simulink model "restart_lv1"  (Simulink 7.1)
settings: Solver=ode3  StartTime=0.0  StopTime=100  FixedStep=0.01  RelTol=1e-3
undefined symbols (not defined in the file or in its folder): fcn
libraries: DRlib x1
settings Model: Creator=lv  LastModifiedBy=lv

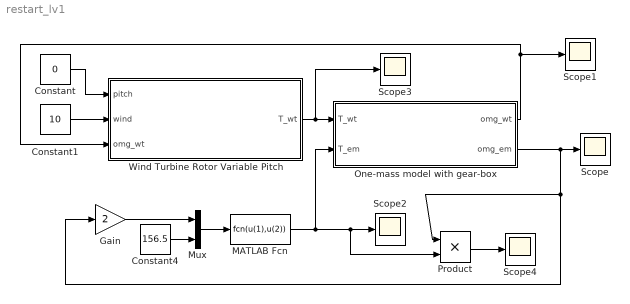
== system restart_lv1 ==
  Constant : Constant  Value=0  OutDataType=sfix(16)  OutScaling=2^0
  Constant1 : Constant  Value=10  OutDataType=sfix(16)  OutScaling=2^0
  Constant4 : Constant  Value=156.5  OutDataType=sfix(16)  OutScaling=2^0
  Gain : Gain  Gain=2  ParameterDataType=sfix(16)  ParameterScaling=2^0  OutDataType=sfix(16)  OutScaling=2^0
  MATLAB Fcn : MATLABFcn  MATLABFcn=fcn(u(1),u(2))  Output1D=off
  Mux : Mux  Inputs=2
  One-mass model with gear-box : Subsystem  AncestorBlock=wt_blockset_v3/Mechanical Components/One-mass model with gear-box  mask(Simple Gearbox){Jem=90, Jwt=49.5e5, K=83.531, init_speed=1.87355}
      mask prompts: Jem "Electric machinery - Moment of inertia [kg m2]"; Jwt "Wind turbine rotor - Moment of inertia [kg*m2]"; K "Gearbox ratio"; init_speed "Initial condition [omg_wt (rad/sec)]"
      mask init:
      | J=Jem*K^2+Jwt;
      mask Display: disp('E M\nGear box')
  Product : Product  OutDataType=sfix(16)  OutScaling=2^0  RndMeth=Zero
  Scope{,1..4} (5 alike) : Scope
      Scope settings: YMin=157.524  YMax=157.524
      Scope1 settings: YMin=1.77385  YMax=1.96057
      Scope2 settings: YMin=72407.5  YMax=72407.5  SaveName=ScopeData2
      Scope3 settings: YMin=5.74586e+006  YMax=6.35068e+006  SaveName=ScopeData3
      Scope4 settings: YMin=1.06296e+007  YMax=1.17485e+007  SaveName=ScopeData6
  Wind Turbine Rotor Variable Pitch : Subsystem  AncestorBlock=|  mask(Aerodynamic model for wind turbine){R=40, ro_air=1.25, cut_in=3, cut_out=25, Tact=0}
      | wt_blockset_v3/Mechanical
      | Components/Wind Turbine Rotor
      | Variable Pitch
      mask prompts: R "Blade radius [m]"; ro_air "Air density [kg m3]"; cut_in "Cut in speed [m/sec]"; cut_out "Cut out speed [m/sec]"; Tact "Time constant for pitch actuator [sec]"
      mask init:
      | load cp_cq;
      | Ctorque=cq(2:5:102,2:5:182);
      | clear Cp cq
      mask Display: plot(20,0,120,200,[45,35,35,45,75,75,45],[85,92,108,115,115,85,85],[55,50,70,65],[115,180,190,115],[55,50,70,65],[85,10,20,85],[75,85],[102,102],[75,85],[98,98],[105,85,85,105],[80,85,115,120])
  wires:
  Wind Turbine Rotor Variable Pitch/1(T_wt) -> One-mass model with gear-box/1(T_wt), Scope3/1
  MATLAB Fcn/1 -> One-mass model with gear-box/2(T_em), Scope2/1, Product/2
  One-mass model with gear-box/1(omg_wt) -> Wind Turbine Rotor Variable Pitch/3(omg_wt), Scope1/1
  Constant/1 -> Wind Turbine Rotor Variable Pitch/1(pitch)
  Constant1/1 -> Wind Turbine Rotor Variable Pitch/2(wind)
  One-mass model with gear-box/2(omg_em) -> Scope/1, Product/1, Gain/1
  Product/1 -> Scope4/1
  Mux/1 -> MATLAB Fcn/1
  Constant4/1 -> Mux/2
  Gain/1 -> Mux/1

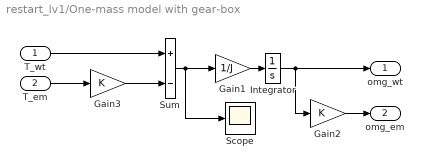
== system restart_lv1/One-mass model with gear-box ==
  T_wt : Inport  OutDataType=sfix(16)  OutScaling=2^0
  T_em : Inport  Port=2  OutDataType=sfix(16)  OutScaling=2^0
  Gain1 : Gain  Gain=1/J  ParameterDataType=sfix(16)  ParameterScaling=2^0  OutDataType=sfix(16)  OutScaling=2^0  SaturateOnIntegerOverflow=on  OutDataTypeStr=Inherit: Same as input  ParamDataTypeStr=Inherit: Same as input
  Gain2 : Gain  Gain=K  ParameterDataType=sfix(16)  ParameterScaling=2^0  OutDataType=sfix(16)  OutScaling=2^0  SaturateOnIntegerOverflow=on  OutDataTypeStr=Inherit: Same as input  ParamDataTypeStr=Inherit: Same as input
  Gain3 : Gain  Gain=K  ParameterDataType=sfix(16)  ParameterScaling=2^0  OutDataType=sfix(16)  OutScaling=2^0  SaturateOnIntegerOverflow=on  OutDataTypeStr=Inherit: Same as input  ParamDataTypeStr=Inherit: Same as input
  Integrator : Integrator  InitialCondition=init_speed  UpperSaturationLimit=0.95*2*pi*60  LowerSaturationLimit=0
  Scope : Scope
      settings: YMin=-3.32483e-008  YMax=-3.00817e-008  SaveName=ScopeData5
  Sum : Sum  Inputs=+-  OutDataType=sfix(16)  OutScaling=2^0  SaturateOnIntegerOverflow=on  InputSameDT=on  OutDataTypeStr=Inherit: Same as first input
  omg_wt : Outport  OutDataType=sfix(16)  OutScaling=2^0  InitialOutput=0
  omg_em : Outport  Port=2  OutDataType=sfix(16)  OutScaling=2^0  InitialOutput=0
  wires:
  Gain3/1 -> Sum/2
  Gain2/1 -> omg_em/1
  Integrator/1 -> Gain2/1, omg_wt/1
  T_wt/1 -> Sum/1
  T_em/1 -> Gain3/1
  Sum/1 -> Gain1/1, Scope/1
  Gain1/1 -> Integrator/1

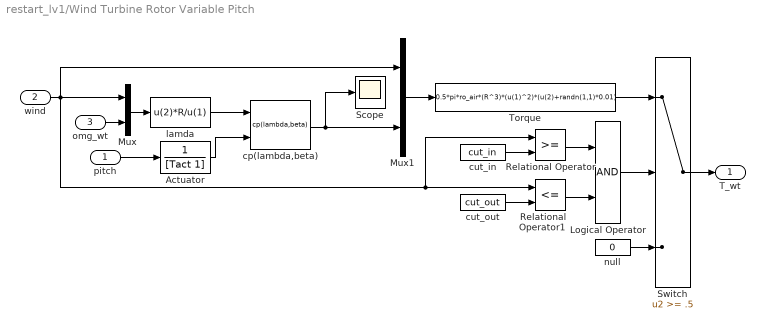
== system restart_lv1/Wind Turbine Rotor Variable Pitch ==
  pitch : Inport  OutDataType=sfix(16)  OutScaling=2^0
  wind : Inport  Port=2  OutDataType=sfix(16)  OutScaling=2^0
  omg_wt : Inport  Port=3  OutDataType=sfix(16)  OutScaling=2^0
  Actuator : TransferFcn  Denominator=[Tact 1]
  Logical Operator : Logic
  Mux : Mux  Inputs=2
  Mux1 : Mux  Inputs=2
  Relational Operator : RelationalOperator  InputSameDT=on
  Relational Operator1 : RelationalOperator  Operator=<=  InputSameDT=on
  Scope : Scope
      settings: YMin=0.447099  YMax=0.494163  SaveName=ScopeData4
  Switch : Switch  Threshold=.5  SaturateOnIntegerOverflow=on  InputSameDT=on
  Torque : Fcn  Expr=0.5*pi*ro_air*(R^3)*(u(1)^2)*(u(2)+randn(1,1)*0.01)
  cp(lambda,beta) : DRlib/Wind Generation/Wind Turbine/cp(lambda,beta)  SystemSampleTime=-1
  cut_in : Constant  Value=cut_in  OutDataType=sfix(16)  OutScaling=2^0
  cut_out : Constant  Value=cut_out  OutDataType=sfix(16)  OutScaling=2^0
  lamda : Fcn  Expr=u(2)*R/u(1)
  null : Constant  Value=0  OutDataType=sfix(16)  OutScaling=2^0
  T_wt : Outport  OutDataType=sfix(16)  OutScaling=2^0
  wires:
  Actuator/1 -> cp(lambda,beta)/2
  Mux/1 -> lamda/1
  Mux1/1 -> Torque/1
  omg_wt/1 -> Mux/2
  cut_in/1 -> Relational Operator/2
  cut_out/1 -> Relational Operator1/2
  Relational Operator1/1 -> Logical Operator/2
  Relational Operator/1 -> Logical Operator/1
  Switch/1 -> T_wt/1
  Torque/1 -> Switch/1
  null/1 -> Switch/3
  Logical Operator/1 -> Switch/2
  wind/1 -> Mux/1, Relational Operator/1, Relational Operator1/1, Mux1/1
  cp(lambda,beta)/1 -> Mux1/2, Scope/1
  lamda/1 -> cp(lambda,beta)/1
  pitch/1 -> Actuator/1
